simulink model "frbd_64ch_600mhz2"  (R2013b)
settings: Solver=FixedStepDiscrete  SolverMode=SingleTasking  StartTime=0.0  StopTime=10.0  RelTol=1e-3
undefined symbols (not defined in the file or in its folder): pfb_coeff_gen_calc
libraries: xbsIndex_r4 x13876, casper_library_misc x58, casper_library_delays x32, dspsigops x16, casper_library_pfbs x2, xps_library x1
(part 16 of 138)

== system frbd_64ch_600mhz2/ACC7/mem ==
  note: Undo address
      | manipulation for
      | simulated data
  note: Undo data manipulation on way in and redo on way out for simulated data
  In1 : Inport
  In2 : Inport  Port=2
  In3 : Inport  Port=3
  Disregard Subsystem : xbsIndex_r4/Disregard Subsystem  Tag=discardX  block_type=disregard
  calc_add : Subsystem  mask{data_width=32, addr_width=10, sample_rate=sample_rate}
      mask prompts: data_width "data width"; addr_width "address width"; sample_rate "sample rate"
  ram : xbsIndex_r4/Single Port RAM  depth=2^addr_width  initVector=init_vals  distributed_mem=Block RAM  write_mode=Read After Write  rst=off  init_reg=0  en=off  latency=3  dbl_ovrd=off  optimize=Area  block_type=spram
  sim_addr : xbsIndex_r4/Gateway In  gui_display_data_type=Fixed-point  arith_type=Unsigned  n_bits=addr_width  bin_pt=0  preci_type=Single  exp_width=8  frac_width=24  quantization=Truncate  overflow=Wrap  period=sample_rate  dbl_ovrd=off  timing_constraint=None  locs_specified=off  LOCs={}  UseAsADC=off  ADCChannel='1'  inherit_from_input=off  hdl_port=on  block_type=gatewayin
      settings: infoedit="Gateway in block.  Converts inputs of type Simulink integer, double and fixed point to  Xilinx fixed point type.<br><br>Hardware notes:  In hardware these blocks become top level input ports."  xl_area=[0, 0, 0, 0, 0, 0, 0]  sginterface={'Nallatech'=>{'xdspkit'=>{'non_memory_mapped_port'=>'sim_addr'}},'Xilinx'=>{'jtaghwcosim'=>{'non_memory_mapped_port'=>'sim_addr'},'xdspkit'=>{'non_memory_mapped_port'=>'sim_addr'}}}
  sim_data_in : xbsIndex_r4/Gateway In  gui_display_data_type=Fixed-point  arith_type=Unsigned  n_bits=32  bin_pt=0  preci_type=Single  exp_width=8  frac_width=24  quantization=Truncate  overflow=Wrap  period=sample_rate  dbl_ovrd=off  timing_constraint=None  locs_specified=off  LOCs={}  UseAsADC=off  ADCChannel='1'  inherit_from_input=off  hdl_port=on  block_type=gatewayin
      settings: xl_area=[0, 0, 0, 0, 0, 0, 0]  sginterface={'Nallatech'=>{'xdspkit'=>{'non_memory_mapped_port'=>'sim_data_in'}},'Xilinx'=>{'jtaghwcosim'=>{'non_memory_mapped_port'=>'sim_data_in'},'xdspkit'=>{'non_memory_mapped_port'=>'sim_data_in'}}}
  sim_data_out : xbsIndex_r4/Gateway Out  inherit_from_input=off  hdl_port=on  timing_constraint=None  locs_specified=off  LOCs={'B21','B22','A22','B23','B19','C19','A20','A21','A23','B24','A24','A25','E18','D18','C18','B18'}  UseAsDAC=off  DACChannel='1'  block_type=gatewayout
      settings: infoedit="Gateway out block.  Converts Xilinx fixed point inputs into ouputs of type Simulink integer, double, or fixed point.<P><P>Hardware notes:  In hardware these blocks become top level output ports or are discarded, depending on how they are configured."  xl_area=[0, 0, 0, 0, 0, 0, 0]  sginterface={'Nallatech'=>{'xdspkit'=>{'non_memory_mapped_port'=>'sim_data_out'}},'Xilinx'=>{'jtaghwcosim'=>{'non_memory_mapped_port'=>'sim_data_out'},'xdspkit'=>{'non_memory_mapped_port'=>'sim_data_out'}}}
  sim_munge_in : Subsystem  AncestorBlock=casper_library_flow_control/munge  mask(munge){divisions=1, div_size=32, order=[0], arith_type_out=Unsigned, bin_pt_out=0}
      mask prompts: divisions "Number of divisions"; div_size "Division size (bits)"; order "Division packing order"; arith_type_out "Output arithmetic type"; bin_pt_out "Output binary point"
      mask help: Splits an input bus into the specified number of divisions and then recombines them in the order specified (most significant division = 0,least = number divisions-1)
      mask init:
      | munge_init(gcb, ...
      |     'divisions', divisions, ...
      |     'div_size', div_size, ...
      |     'order', order, ...
      |     'arith_type_out', arith_type_out, ...
      |     'bin_pt_out', bin_pt_out);
      settings: AttributesFormatString=|
      | split:32
      | join:0
      | Unsigned [32,0]
      mask TypeOptions arith_type_out: Unsigned | Signed  (2's comp) | Floating-point
  sim_munge_out : Subsystem  AncestorBlock=casper_library_flow_control/munge  mask(munge){divisions=1, div_size=32, order=[0], arith_type_out=Unsigned, bin_pt_out=0}
      mask prompts: divisions "Number of divisions"; div_size "Division size (bits)"; order "Division packing order"; arith_type_out "Output arithmetic type"; bin_pt_out "Output binary point"
      mask help: Splits an input bus into the specified number of divisions and then recombines them in the order specified (most significant division = 0,least = number divisions-1)
      mask init:
      | munge_init(gcb, ...
      |     'divisions', divisions, ...
      |     'div_size', div_size, ...
      |     'order', order, ...
      |     'arith_type_out', arith_type_out, ...
      |     'bin_pt_out', bin_pt_out);
      settings: AttributesFormatString=|
      | split:32
      | join:0
      | Unsigned [32,0]
      mask TypeOptions arith_type_out: Unsigned | Signed  (2's comp) | Floating-point
  sim_we : xbsIndex_r4/Gateway In  gui_display_data_type=Fixed-point  arith_type=Boolean  n_bits=1  bin_pt=0  preci_type=Single  exp_width=8  frac_width=24  quantization=Truncate  overflow=Wrap  period=sample_rate  dbl_ovrd=off  timing_constraint=None  locs_specified=off  LOCs={}  UseAsADC=off  ADCChannel='1'  inherit_from_input=off  hdl_port=on  block_type=gatewayin
      settings: infoedit="Gateway in block.  Converts inputs of type Simulink integer, double and fixed point to  Xilinx fixed point type.<br><br>Hardware notes:  In hardware these blocks become top level input ports."  xl_area=[0, 0, 0, 0, 0, 0, 0]  sginterface={'Nallatech'=>{'xdspkit'=>{'non_memory_mapped_port'=>'sim_we'}},'Xilinx'=>{'jtaghwcosim'=>{'non_memory_mapped_port'=>'sim_we'},'xdspkit'=>{'non_memory_mapped_port'=>'sim_we'}}}
  Out1 : Outport
  wires:
  sim_munge_in/1(dout) -> ram/2
  ram/1 -> sim_munge_out/1(din)
  sim_we/1 -> ram/3
  sim_data_in/1 -> sim_munge_in/1(din)
  sim_addr/1 -> calc_add/1(in)
  In3/1 -> sim_we/1
  sim_data_out/1 -> Out1/1
  In2/1 -> sim_data_in/1
  In1/1 -> sim_addr/1
  sim_munge_out/1(dout) -> sim_data_out/1
  calc_add/1(out) -> ram/1

== system frbd_64ch_600mhz2/ACC7/munge_in ==
  din : Inport
  reinterpret_out : xbsIndex_r4/Reinterpret  force_arith_type=on  arith_type=Unsigned  force_bin_pt=on  bin_pt=0  block_type=reinterpret
  dout : Outport
  wires:
  reinterpret_out/1 -> dout/1
  din/1 -> reinterpret_out/1

== system frbd_64ch_600mhz2/ACC7/munge_out ==
  din : Inport
  reinterpret_out : xbsIndex_r4/Reinterpret  force_arith_type=on  arith_type=Unsigned  force_bin_pt=on  bin_pt=0  block_type=reinterpret
  dout : Outport
  wires:
  reinterpret_out/1 -> dout/1
  din/1 -> reinterpret_out/1

== system frbd_64ch_600mhz2/ACC8/calc_add ==
  note: Use behavioural HDL
      | so that gets optimised
      | to minimum logic
  note: If reading/writing words
      | smaller than 32 bits,
      | change address so
      | that addressing is
      | big endian instead of
      | little, otherwise
      | pass through
  in : Inport
  add_sub : xbsIndex_r4/AddSub  mode=Subtraction  use_carryin=off  use_carryout=off  en=off  latency=0  precision=User Defined  arith_type=Unsigned  n_bits=max(1, log2(32/data_width))  bin_pt=0  quantization=Truncate  overflow=Wrap  dbl_ovrd=off  use_behavioral_HDL=on  hw_selection=Fabric  pipelined=off  block_type=addsub
  concat : xbsIndex_r4/Concat  num_inputs=2  dbl_ovrd=off  block_type=concat
  const : xbsIndex_r4/Constant  const=max(0, 32/data_width-1)  gui_display_data_type=Fixed-point  arith_type=Unsigned  n_bits=max(1, log2(32/data_width))  bin_pt=0  preci_type=Single  exp_width=8  frac_width=24  explicit_period=on  period=sample_rate  equ=P=C  opselect=C  inp2=PCIN>>17  opr=+  inp1=P  carry=CIN  dbl_ovrd=off  block_type=constant
      settings: block_version=11.4
  convert_addr : xbsIndex_r4/Convert  gui_display_data_type=Fixed-point  arith_type=Unsigned  n_bits=addr_width  bin_pt=0  float_type=Single  exp_bits=8  fraction_bits=24  quantization=Truncate  overflow=Wrap  en=off  latency=0  dbl_ovrd=off  pipeline=off  block_type=convert
      settings: xl_area=[0, 0, 0, 0, 0, 0, 0]
  lsw : xbsIndex_r4/Slice  nbits=max(1, log2(32/data_width))  boolean_output=off  mode=Lower Bit Location + Width  bit1=0  base1=MSB of Input  bit0=0  base0=LSB of Input  dbl_ovrd=off  block_type=slice
  manipulate : xbsIndex_r4/Constant  const=min(1, floor(32/data_width) - 1)  gui_display_data_type=Fixed-point  arith_type=Unsigned  n_bits=1  bin_pt=0  preci_type=Single  exp_width=8  frac_width=24  explicit_period=on  period=sample_rate  equ=P=C  opselect=C  inp2=PCIN>>17  opr=+  inp1=P  carry=CIN  dbl_ovrd=off  block_type=constant
      settings: block_version=11.4
  msw : xbsIndex_r4/Slice  nbits=addr_width - max(1, log2(32/data_width))  boolean_output=off  mode=Upper Bit Location + Width  bit1=0  base1=MSB of Input  bit0=0  base0=LSB of Input  dbl_ovrd=off  block_type=slice
  mux : xbsIndex_r4/Mux  inputs=2  en=off  latency=0  precision=Full  arith_type=Unsigned  n_bits=16  bin_pt=14  quantization=Truncate  overflow=Wrap  dbl_ovrd=off  block_type=mux
      settings: block_version=11.4
  out : Outport
  wires:
  convert_addr/1 -> mux/2, msw/1, lsw/1
  const/1 -> add_sub/1
  lsw/1 -> add_sub/2
  mux/1 -> out/1
  manipulate/1 -> mux/1
  concat/1 -> mux/3
  msw/1 -> concat/1
  add_sub/1 -> concat/2
  in/1 -> convert_addr/1

== system frbd_64ch_600mhz2/ACC8/mem ==
  note: Undo data manipulation on way in and redo on way out for simulated data
  note: Undo address
      | manipulation for
      | simulated data
  In1 : Inport
  In2 : Inport  Port=2
  In3 : Inport  Port=3
  Disregard Subsystem : xbsIndex_r4/Disregard Subsystem  Tag=discardX  block_type=disregard
  calc_add : Subsystem  mask{data_width=32, addr_width=10, sample_rate=sample_rate}
      mask prompts: data_width "data width"; addr_width "address width"; sample_rate "sample rate"
  ram : xbsIndex_r4/Single Port RAM  depth=2^addr_width  initVector=init_vals  distributed_mem=Block RAM  write_mode=Read After Write  rst=off  init_reg=0  en=off  latency=3  dbl_ovrd=off  optimize=Area  block_type=spram
  sim_addr : xbsIndex_r4/Gateway In  gui_display_data_type=Fixed-point  arith_type=Unsigned  n_bits=addr_width  bin_pt=0  preci_type=Single  exp_width=8  frac_width=24  quantization=Truncate  overflow=Wrap  period=sample_rate  dbl_ovrd=off  timing_constraint=None  locs_specified=off  LOCs={}  UseAsADC=off  ADCChannel='1'  inherit_from_input=off  hdl_port=on  block_type=gatewayin
      settings: infoedit="Gateway in block.  Converts inputs of type Simulink integer, double and fixed point to  Xilinx fixed point type.<br><br>Hardware notes:  In hardware these blocks become top level input ports."  xl_area=[0, 0, 0, 0, 0, 0, 0]  sginterface={'Nallatech'=>{'xdspkit'=>{'non_memory_mapped_port'=>'sim_addr'}},'Xilinx'=>{'jtaghwcosim'=>{'non_memory_mapped_port'=>'sim_addr'},'xdspkit'=>{'non_memory_mapped_port'=>'sim_addr'}}}
  sim_data_in : xbsIndex_r4/Gateway In  gui_display_data_type=Fixed-point  arith_type=Unsigned  n_bits=32  bin_pt=0  preci_type=Single  exp_width=8  frac_width=24  quantization=Truncate  overflow=Wrap  period=sample_rate  dbl_ovrd=off  timing_constraint=None  locs_specified=off  LOCs={}  UseAsADC=off  ADCChannel='1'  inherit_from_input=off  hdl_port=on  block_type=gatewayin
      settings: xl_area=[0, 0, 0, 0, 0, 0, 0]  sginterface={'Nallatech'=>{'xdspkit'=>{'non_memory_mapped_port'=>'sim_data_in'}},'Xilinx'=>{'jtaghwcosim'=>{'non_memory_mapped_port'=>'sim_data_in'},'xdspkit'=>{'non_memory_mapped_port'=>'sim_data_in'}}}
  sim_data_out : xbsIndex_r4/Gateway Out  inherit_from_input=off  hdl_port=on  timing_constraint=None  locs_specified=off  LOCs={'B21','B22','A22','B23','B19','C19','A20','A21','A23','B24','A24','A25','E18','D18','C18','B18'}  UseAsDAC=off  DACChannel='1'  block_type=gatewayout
      settings: infoedit="Gateway out block.  Converts Xilinx fixed point inputs into ouputs of type Simulink integer, double, or fixed point.<P><P>Hardware notes:  In hardware these blocks become top level output ports or are discarded, depending on how they are configured."  xl_area=[0, 0, 0, 0, 0, 0, 0]  sginterface={'Nallatech'=>{'xdspkit'=>{'non_memory_mapped_port'=>'sim_data_out'}},'Xilinx'=>{'jtaghwcosim'=>{'non_memory_mapped_port'=>'sim_data_out'},'xdspkit'=>{'non_memory_mapped_port'=>'sim_data_out'}}}
  sim_munge_in : Subsystem  AncestorBlock=casper_library_flow_control/munge  mask(munge){divisions=1, div_size=32, order=[0], arith_type_out=Unsigned, bin_pt_out=0}
      mask prompts: divisions "Number of divisions"; div_size "Division size (bits)"; order "Division packing order"; arith_type_out "Output arithmetic type"; bin_pt_out "Output binary point"
      mask help: Splits an input bus into the specified number of divisions and then recombines them in the order specified (most significant division = 0,least = number divisions-1)
      mask init:
      | munge_init(gcb, ...
      |     'divisions', divisions, ...
      |     'div_size', div_size, ...
      |     'order', order, ...
      |     'arith_type_out', arith_type_out, ...
      |     'bin_pt_out', bin_pt_out);
      settings: AttributesFormatString=|
      | split:32
      | join:0
      | Unsigned [32,0]
      mask TypeOptions arith_type_out: Unsigned | Signed  (2's comp) | Floating-point
  sim_munge_out : Subsystem  AncestorBlock=casper_library_flow_control/munge  mask(munge){divisions=1, div_size=32, order=[0], arith_type_out=Unsigned, bin_pt_out=0}
      mask prompts: divisions "Number of divisions"; div_size "Division size (bits)"; order "Division packing order"; arith_type_out "Output arithmetic type"; bin_pt_out "Output binary point"
      mask help: Splits an input bus into the specified number of divisions and then recombines them in the order specified (most significant division = 0,least = number divisions-1)
      mask init:
      | munge_init(gcb, ...
      |     'divisions', divisions, ...
      |     'div_size', div_size, ...
      |     'order', order, ...
      |     'arith_type_out', arith_type_out, ...
      |     'bin_pt_out', bin_pt_out);
      settings: AttributesFormatString=|
      | split:32
      | join:0
      | Unsigned [32,0]
      mask TypeOptions arith_type_out: Unsigned | Signed  (2's comp) | Floating-point
  sim_we : xbsIndex_r4/Gateway In  gui_display_data_type=Fixed-point  arith_type=Boolean  n_bits=1  bin_pt=0  preci_type=Single  exp_width=8  frac_width=24  quantization=Truncate  overflow=Wrap  period=sample_rate  dbl_ovrd=off  timing_constraint=None  locs_specified=off  LOCs={}  UseAsADC=off  ADCChannel='1'  inherit_from_input=off  hdl_port=on  block_type=gatewayin
      settings: infoedit="Gateway in block.  Converts inputs of type Simulink integer, double and fixed point to  Xilinx fixed point type.<br><br>Hardware notes:  In hardware these blocks become top level input ports."  xl_area=[0, 0, 0, 0, 0, 0, 0]  sginterface={'Nallatech'=>{'xdspkit'=>{'non_memory_mapped_port'=>'sim_we'}},'Xilinx'=>{'jtaghwcosim'=>{'non_memory_mapped_port'=>'sim_we'},'xdspkit'=>{'non_memory_mapped_port'=>'sim_we'}}}
  Out1 : Outport
  wires:
  calc_add/1(out) -> ram/1
  sim_munge_out/1(dout) -> sim_data_out/1
  In1/1 -> sim_addr/1
  In2/1 -> sim_data_in/1
  sim_data_out/1 -> Out1/1
  In3/1 -> sim_we/1
  sim_addr/1 -> calc_add/1(in)
  sim_data_in/1 -> sim_munge_in/1(din)
  sim_we/1 -> ram/3
  ram/1 -> sim_munge_out/1(din)
  sim_munge_in/1(dout) -> ram/2

== system frbd_64ch_600mhz2/ACC8/munge_in ==
  din : Inport
  reinterpret_out : xbsIndex_r4/Reinterpret  force_arith_type=on  arith_type=Unsigned  force_bin_pt=on  bin_pt=0  block_type=reinterpret
  dout : Outport
  wires:
  din/1 -> reinterpret_out/1
  reinterpret_out/1 -> dout/1

== system frbd_64ch_600mhz2/ACC8/munge_out ==
  din : Inport
  reinterpret_out : xbsIndex_r4/Reinterpret  force_arith_type=on  arith_type=Unsigned  force_bin_pt=on  bin_pt=0  block_type=reinterpret
  dout : Outport
  wires:
  din/1 -> reinterpret_out/1
  reinterpret_out/1 -> dout/1

== system frbd_64ch_600mhz2/ACC9/calc_add ==
  note: Use behavioural HDL
      | so that gets optimised
      | to minimum logic
  note: If reading/writing words
      | smaller than 32 bits,
      | change address so
      | that addressing is
      | big endian instead of
      | little, otherwise
      | pass through
  in : Inport
  add_sub : xbsIndex_r4/AddSub  mode=Subtraction  use_carryin=off  use_carryout=off  en=off  latency=0  precision=User Defined  arith_type=Unsigned  n_bits=max(1, log2(32/data_width))  bin_pt=0  quantization=Truncate  overflow=Wrap  dbl_ovrd=off  use_behavioral_HDL=on  hw_selection=Fabric  pipelined=off  block_type=addsub
  concat : xbsIndex_r4/Concat  num_inputs=2  dbl_ovrd=off  block_type=concat
  const : xbsIndex_r4/Constant  const=max(0, 32/data_width-1)  gui_display_data_type=Fixed-point  arith_type=Unsigned  n_bits=max(1, log2(32/data_width))  bin_pt=0  preci_type=Single  exp_width=8  frac_width=24  explicit_period=on  period=sample_rate  equ=P=C  opselect=C  inp2=PCIN>>17  opr=+  inp1=P  carry=CIN  dbl_ovrd=off  block_type=constant
      settings: block_version=11.4
  convert_addr : xbsIndex_r4/Convert  gui_display_data_type=Fixed-point  arith_type=Unsigned  n_bits=addr_width  bin_pt=0  float_type=Single  exp_bits=8  fraction_bits=24  quantization=Truncate  overflow=Wrap  en=off  latency=0  dbl_ovrd=off  pipeline=off  block_type=convert
      settings: xl_area=[0, 0, 0, 0, 0, 0, 0]
  lsw : xbsIndex_r4/Slice  nbits=max(1, log2(32/data_width))  boolean_output=off  mode=Lower Bit Location + Width  bit1=0  base1=MSB of Input  bit0=0  base0=LSB of Input  dbl_ovrd=off  block_type=slice
  manipulate : xbsIndex_r4/Constant  const=min(1, floor(32/data_width) - 1)  gui_display_data_type=Fixed-point  arith_type=Unsigned  n_bits=1  bin_pt=0  preci_type=Single  exp_width=8  frac_width=24  explicit_period=on  period=sample_rate  equ=P=C  opselect=C  inp2=PCIN>>17  opr=+  inp1=P  carry=CIN  dbl_ovrd=off  block_type=constant
      settings: block_version=11.4
  msw : xbsIndex_r4/Slice  nbits=addr_width - max(1, log2(32/data_width))  boolean_output=off  mode=Upper Bit Location + Width  bit1=0  base1=MSB of Input  bit0=0  base0=LSB of Input  dbl_ovrd=off  block_type=slice
  mux : xbsIndex_r4/Mux  inputs=2  en=off  latency=0  precision=Full  arith_type=Unsigned  n_bits=16  bin_pt=14  quantization=Truncate  overflow=Wrap  dbl_ovrd=off  block_type=mux
      settings: block_version=11.4
  out : Outport
  wires:
  convert_addr/1 -> mux/2, msw/1, lsw/1
  const/1 -> add_sub/1
  lsw/1 -> add_sub/2
  mux/1 -> out/1
  manipulate/1 -> mux/1
  concat/1 -> mux/3
  msw/1 -> concat/1
  add_sub/1 -> concat/2
  in/1 -> convert_addr/1

== system frbd_64ch_600mhz2/ACC9/mem ==
  note: Undo data manipulation on way in and redo on way out for simulated data
  note: Undo address
      | manipulation for
      | simulated data
  In1 : Inport
  In2 : Inport  Port=2
  In3 : Inport  Port=3
  Disregard Subsystem : xbsIndex_r4/Disregard Subsystem  Tag=discardX  block_type=disregard
  calc_add : Subsystem  mask{data_width=32, addr_width=10, sample_rate=sample_rate}
      mask prompts: data_width "data width"; addr_width "address width"; sample_rate "sample rate"
  ram : xbsIndex_r4/Single Port RAM  depth=2^addr_width  initVector=init_vals  distributed_mem=Block RAM  write_mode=Read After Write  rst=off  init_reg=0  en=off  latency=3  dbl_ovrd=off  optimize=Area  block_type=spram
  sim_addr : xbsIndex_r4/Gateway In  gui_display_data_type=Fixed-point  arith_type=Unsigned  n_bits=addr_width  bin_pt=0  preci_type=Single  exp_width=8  frac_width=24  quantization=Truncate  overflow=Wrap  period=sample_rate  dbl_ovrd=off  timing_constraint=None  locs_specified=off  LOCs={}  UseAsADC=off  ADCChannel='1'  inherit_from_input=off  hdl_port=on  block_type=gatewayin
      settings: infoedit="Gateway in block.  Converts inputs of type Simulink integer, double and fixed point to  Xilinx fixed point type.<br><br>Hardware notes:  In hardware these blocks become top level input ports."  xl_area=[0, 0, 0, 0, 0, 0, 0]  sginterface={'Nallatech'=>{'xdspkit'=>{'non_memory_mapped_port'=>'sim_addr'}},'Xilinx'=>{'jtaghwcosim'=>{'non_memory_mapped_port'=>'sim_addr'},'xdspkit'=>{'non_memory_mapped_port'=>'sim_addr'}}}
  sim_data_in : xbsIndex_r4/Gateway In  gui_display_data_type=Fixed-point  arith_type=Unsigned  n_bits=32  bin_pt=0  preci_type=Single  exp_width=8  frac_width=24  quantization=Truncate  overflow=Wrap  period=sample_rate  dbl_ovrd=off  timing_constraint=None  locs_specified=off  LOCs={}  UseAsADC=off  ADCChannel='1'  inherit_from_input=off  hdl_port=on  block_type=gatewayin
      settings: xl_area=[0, 0, 0, 0, 0, 0, 0]  sginterface={'Nallatech'=>{'xdspkit'=>{'non_memory_mapped_port'=>'sim_data_in'}},'Xilinx'=>{'jtaghwcosim'=>{'non_memory_mapped_port'=>'sim_data_in'},'xdspkit'=>{'non_memory_mapped_port'=>'sim_data_in'}}}
  sim_data_out : xbsIndex_r4/Gateway Out  inherit_from_input=off  hdl_port=on  timing_constraint=None  locs_specified=off  LOCs={'B21','B22','A22','B23','B19','C19','A20','A21','A23','B24','A24','A25','E18','D18','C18','B18'}  UseAsDAC=off  DACChannel='1'  block_type=gatewayout
      settings: infoedit="Gateway out block.  Converts Xilinx fixed point inputs into ouputs of type Simulink integer, double, or fixed point.<P><P>Hardware notes:  In hardware these blocks become top level output ports or are discarded, depending on how they are configured."  xl_area=[0, 0, 0, 0, 0, 0, 0]  sginterface={'Nallatech'=>{'xdspkit'=>{'non_memory_mapped_port'=>'sim_data_out'}},'Xilinx'=>{'jtaghwcosim'=>{'non_memory_mapped_port'=>'sim_data_out'},'xdspkit'=>{'non_memory_mapped_port'=>'sim_data_out'}}}
  sim_munge_in : Subsystem  AncestorBlock=casper_library_flow_control/munge  mask(munge){divisions=1, div_size=32, order=[0], arith_type_out=Unsigned, bin_pt_out=0}
      mask prompts: divisions "Number of divisions"; div_size "Division size (bits)"; order "Division packing order"; arith_type_out "Output arithmetic type"; bin_pt_out "Output binary point"
      mask help: Splits an input bus into the specified number of divisions and then recombines them in the order specified (most significant division = 0,least = number divisions-1)
      mask init:
      | munge_init(gcb, ...
      |     'divisions', divisions, ...
      |     'div_size', div_size, ...
      |     'order', order, ...
      |     'arith_type_out', arith_type_out, ...
      |     'bin_pt_out', bin_pt_out);
      settings: AttributesFormatString=|
      | split:32
      | join:0
      | Unsigned [32,0]
      mask TypeOptions arith_type_out: Unsigned | Signed  (2's comp) | Floating-point
  sim_munge_out : Subsystem  AncestorBlock=casper_library_flow_control/munge  mask(munge){divisions=1, div_size=32, order=[0], arith_type_out=Unsigned, bin_pt_out=0}
      mask prompts: divisions "Number of divisions"; div_size "Division size (bits)"; order "Division packing order"; arith_type_out "Output arithmetic type"; bin_pt_out "Output binary point"
      mask help: Splits an input bus into the specified number of divisions and then recombines them in the order specified (most significant division = 0,least = number divisions-1)
      mask init:
      | munge_init(gcb, ...
      |     'divisions', divisions, ...
      |     'div_size', div_size, ...
      |     'order', order, ...
      |     'arith_type_out', arith_type_out, ...
      |     'bin_pt_out', bin_pt_out);
      settings: AttributesFormatString=|
      | split:32
      | join:0
      | Unsigned [32,0]
      mask TypeOptions arith_type_out: Unsigned | Signed  (2's comp) | Floating-point
  sim_we : xbsIndex_r4/Gateway In  gui_display_data_type=Fixed-point  arith_type=Boolean  n_bits=1  bin_pt=0  preci_type=Single  exp_width=8  frac_width=24  quantization=Truncate  overflow=Wrap  period=sample_rate  dbl_ovrd=off  timing_constraint=None  locs_specified=off  LOCs={}  UseAsADC=off  ADCChannel='1'  inherit_from_input=off  hdl_port=on  block_type=gatewayin
      settings: infoedit="Gateway in block.  Converts inputs of type Simulink integer, double and fixed point to  Xilinx fixed point type.<br><br>Hardware notes:  In hardware these blocks become top level input ports."  xl_area=[0, 0, 0, 0, 0, 0, 0]  sginterface={'Nallatech'=>{'xdspkit'=>{'non_memory_mapped_port'=>'sim_we'}},'Xilinx'=>{'jtaghwcosim'=>{'non_memory_mapped_port'=>'sim_we'},'xdspkit'=>{'non_memory_mapped_port'=>'sim_we'}}}
  Out1 : Outport
  wires:
  calc_add/1(out) -> ram/1
  sim_munge_out/1(dout) -> sim_data_out/1
  In1/1 -> sim_addr/1
  In2/1 -> sim_data_in/1
  sim_data_out/1 -> Out1/1
  In3/1 -> sim_we/1
  sim_addr/1 -> calc_add/1(in)
  sim_data_in/1 -> sim_munge_in/1(din)
  sim_we/1 -> ram/3
  ram/1 -> sim_munge_out/1(din)
  sim_munge_in/1(dout) -> ram/2

== system frbd_64ch_600mhz2/ACC9/munge_in ==
  din : Inport
  reinterpret_out : xbsIndex_r4/Reinterpret  force_arith_type=on  arith_type=Unsigned  force_bin_pt=on  bin_pt=0  block_type=reinterpret
  dout : Outport
  wires:
  din/1 -> reinterpret_out/1
  reinterpret_out/1 -> dout/1

== system frbd_64ch_600mhz2/ACC9/munge_out ==
  din : Inport
  reinterpret_out : xbsIndex_r4/Reinterpret  force_arith_type=on  arith_type=Unsigned  force_bin_pt=on  bin_pt=0  block_type=reinterpret
  dout : Outport
  wires:
  din/1 -> reinterpret_out/1
  reinterpret_out/1 -> dout/1

== system frbd_64ch_600mhz2/Parallel_Dedispersor_v1/Dedispersor_v2_1 ==
  Data : Inport
  Valid : Inport  Port=2
  Counter : xbsIndex_r4/Counter  cnt_type=Free Running  cnt_to=Inf  operation=Up  start_count=0  cnt_by_val=1  arith_type=Unsigned  n_bits=4  bin_pt=0  load_pin=off  rst=off  en=on  explicit_period=on  period=1  dbl_ovrd=off  use_behavioral_HDL=off  implementation=Fabric  block_type=counter
  Mux : xbsIndex_r4/Mux  inputs=16  en=off  latency=0  precision=Full  arith_type=Unsigned  n_bits=16  bin_pt=14  quantization=Truncate  overflow=Wrap  dbl_ovrd=off  block_type=mux
  detector_block_v2 : Subsystem  AncestorBlock=honestlibrary/detector_block_v2  mask(Basic block for FRB detection){chn=0, lat=1, nbits=4}
      mask prompts: chn "Channel"; lat "Latency"; nbits "Number of Bits (Counter)"
      mask help:
      | Delays a certain channel a number of latency clock cycles, according to the fixed DM table.
      | This version incorporates an internal counter (nbits) to know when store or give a certain value.
      mask init:
      | detector_block_init_v2(gcb,'chn',chn,'lat',lat,'nbits',nbits)
      settings: AttributesFormatString=Channel: 0, Delay: 1
  detector_block_v21 : Subsystem  AncestorBlock=honestlibrary/detector_block_v2  mask(Basic block for FRB detection){chn=1, lat=12, nbits=4}
      mask prompts: chn "Channel"; lat "Latency"; nbits "Number of Bits (Counter)"
      mask help:
      | Delays a certain channel a number of latency clock cycles, according to the fixed DM table.
      | This version incorporates an internal counter (nbits) to know when store or give a certain value.
      mask init:
      | detector_block_init_v2(gcb,'chn',chn,'lat',lat,'nbits',nbits)
      settings: AttributesFormatString=Channel: 1, Delay: 12
  detector_block_v210 : Subsystem  AncestorBlock=honestlibrary/detector_block_v2  mask(Basic block for FRB detection){chn=10, lat=89, nbits=4}
      mask prompts: chn "Channel"; lat "Latency"; nbits "Number of Bits (Counter)"
      mask help:
      | Delays a certain channel a number of latency clock cycles, according to the fixed DM table.
      | This version incorporates an internal counter (nbits) to know when store or give a certain value.
      mask init:
      | detector_block_init_v2(gcb,'chn',chn,'lat',lat,'nbits',nbits)
      settings: AttributesFormatString=Channel: 10, Delay: 89
  detector_block_v211 : Subsystem  AncestorBlock=honestlibrary/detector_block_v2  mask(Basic block for FRB detection){chn=11, lat=95, nbits=4}
      mask prompts: chn "Channel"; lat "Latency"; nbits "Number of Bits (Counter)"
      mask help:
      | Delays a certain channel a number of latency clock cycles, according to the fixed DM table.
      | This version incorporates an internal counter (nbits) to know when store or give a certain value.
      mask init:
      | detector_block_init_v2(gcb,'chn',chn,'lat',lat,'nbits',nbits)
      settings: AttributesFormatString=Channel: 11, Delay: 95
  detector_block_v212 : Subsystem  AncestorBlock=honestlibrary/detector_block_v2  mask(Basic block for FRB detection){chn=12, lat=100, nbits=4}
      mask prompts: chn "Channel"; lat "Latency"; nbits "Number of Bits (Counter)"
      mask help:
      | Delays a certain channel a number of latency clock cycles, according to the fixed DM table.
      | This version incorporates an internal counter (nbits) to know when store or give a certain value.
      mask init:
      | detector_block_init_v2(gcb,'chn',chn,'lat',lat,'nbits',nbits)
      settings: AttributesFormatString=Channel: 12, Delay: 100
  detector_block_v213 : Subsystem  AncestorBlock=honestlibrary/detector_block_v2  mask(Basic block for FRB detection){chn=13, lat=105, nbits=4}
      mask prompts: chn "Channel"; lat "Latency"; nbits "Number of Bits (Counter)"
      mask help:
      | Delays a certain channel a number of latency clock cycles, according to the fixed DM table.
      | This version incorporates an internal counter (nbits) to know when store or give a certain value.
      mask init:
      | detector_block_init_v2(gcb,'chn',chn,'lat',lat,'nbits',nbits)
      settings: AttributesFormatString=Channel: 13, Delay: 105
  detector_block_v214 : Subsystem  AncestorBlock=honestlibrary/detector_block_v2  mask(Basic block for FRB detection){chn=14, lat=110, nbits=4}
      mask prompts: chn "Channel"; lat "Latency"; nbits "Number of Bits (Counter)"
      mask help:
      | Delays a certain channel a number of latency clock cycles, according to the fixed DM table.
      | This version incorporates an internal counter (nbits) to know when store or give a certain value.
      mask init:
      | detector_block_init_v2(gcb,'chn',chn,'lat',lat,'nbits',nbits)
      settings: AttributesFormatString=Channel: 14, Delay: 110
  detector_block_v215 : Subsystem  AncestorBlock=honestlibrary/detector_block_v2  mask(Basic block for FRB detection){chn=15, lat=114, nbits=4}
      mask prompts: chn "Channel"; lat "Latency"; nbits "Number of Bits (Counter)"
      mask help:
      | Delays a certain channel a number of latency clock cycles, according to the fixed DM table.
      | This version incorporates an internal counter (nbits) to know when store or give a certain value.
      mask init:
      | detector_block_init_v2(gcb,'chn',chn,'lat',lat,'nbits',nbits)
      settings: AttributesFormatString=Channel: 15, Delay: 114
  detector_block_v22 : Subsystem  AncestorBlock=honestlibrary/detector_block_v2  mask(Basic block for FRB detection){chn=2, lat=23, nbits=4}
      mask prompts: chn "Channel"; lat "Latency"; nbits "Number of Bits (Counter)"
      mask help:
      | Delays a certain channel a number of latency clock cycles, according to the fixed DM table.
      | This version incorporates an internal counter (nbits) to know when store or give a certain value.
      mask init:
      | detector_block_init_v2(gcb,'chn',chn,'lat',lat,'nbits',nbits)
      settings: AttributesFormatString=Channel: 2, Delay: 23
  detector_block_v23 : Subsystem  AncestorBlock=honestlibrary/detector_block_v2  mask(Basic block for FRB detection){chn=3, lat=34, nbits=4}
      mask prompts: chn "Channel"; lat "Latency"; nbits "Number of Bits (Counter)"
      mask help:
      | Delays a certain channel a number of latency clock cycles, according to the fixed DM table.
      | This version incorporates an internal counter (nbits) to know when store or give a certain value.
      mask init:
      | detector_block_init_v2(gcb,'chn',chn,'lat',lat,'nbits',nbits)
      settings: AttributesFormatString=Channel: 3, Delay: 34
  detector_block_v24 : Subsystem  AncestorBlock=honestlibrary/detector_block_v2  mask(Basic block for FRB detection){chn=4, lat=44, nbits=4}
      mask prompts: chn "Channel"; lat "Latency"; nbits "Number of Bits (Counter)"
      mask help:
      | Delays a certain channel a number of latency clock cycles, according to the fixed DM table.
      | This version incorporates an internal counter (nbits) to know when store or give a certain value.
      mask init:
      | detector_block_init_v2(gcb,'chn',chn,'lat',lat,'nbits',nbits)
      settings: AttributesFormatString=Channel: 4, Delay: 44
  detector_block_v25 : Subsystem  AncestorBlock=honestlibrary/detector_block_v2  mask(Basic block for FRB detection){chn=5, lat=53, nbits=4}
      mask prompts: chn "Channel"; lat "Latency"; nbits "Number of Bits (Counter)"
      mask help:
      | Delays a certain channel a number of latency clock cycles, according to the fixed DM table.
      | This version incorporates an internal counter (nbits) to know when store or give a certain value.
      mask init:
      | detector_block_init_v2(gcb,'chn',chn,'lat',lat,'nbits',nbits)
      settings: AttributesFormatString=Channel: 5, Delay: 53
  detector_block_v26 : Subsystem  AncestorBlock=honestlibrary/detector_block_v2  mask(Basic block for FRB detection){chn=6, lat=61, nbits=4}
      mask prompts: chn "Channel"; lat "Latency"; nbits "Number of Bits (Counter)"
      mask help:
      | Delays a certain channel a number of latency clock cycles, according to the fixed DM table.
      | This version incorporates an internal counter (nbits) to know when store or give a certain value.
      mask init:
      | detector_block_init_v2(gcb,'chn',chn,'lat',lat,'nbits',nbits)
      settings: AttributesFormatString=Channel: 6, Delay: 61
  detector_block_v27 : Subsystem  AncestorBlock=honestlibrary/detector_block_v2  mask(Basic block for FRB detection){chn=7, lat=69, nbits=4}
      mask prompts: chn "Channel"; lat "Latency"; nbits "Number of Bits (Counter)"
      mask help:
      | Delays a certain channel a number of latency clock cycles, according to the fixed DM table.
      | This version incorporates an internal counter (nbits) to know when store or give a certain value.
      mask init:
      | detector_block_init_v2(gcb,'chn',chn,'lat',lat,'nbits',nbits)
      settings: AttributesFormatString=Channel: 7, Delay: 69
  detector_block_v28 : Subsystem  AncestorBlock=honestlibrary/detector_block_v2  mask(Basic block for FRB detection){chn=8, lat=76, nbits=4}
      mask prompts: chn "Channel"; lat "Latency"; nbits "Number of Bits (Counter)"
      mask help:
      | Delays a certain channel a number of latency clock cycles, according to the fixed DM table.
      | This version incorporates an internal counter (nbits) to know when store or give a certain value.
      mask init:
      | detector_block_init_v2(gcb,'chn',chn,'lat',lat,'nbits',nbits)
      settings: AttributesFormatString=Channel: 8, Delay: 76
  detector_block_v29 : Subsystem  AncestorBlock=honestlibrary/detector_block_v2  mask(Basic block for FRB detection){chn=9, lat=83, nbits=4}
      mask prompts: chn "Channel"; lat "Latency"; nbits "Number of Bits (Counter)"
      mask help:
      | Delays a certain channel a number of latency clock cycles, according to the fixed DM table.
      | This version incorporates an internal counter (nbits) to know when store or give a certain value.
      mask init:
      | detector_block_init_v2(gcb,'chn',chn,'lat',lat,'nbits',nbits)
      settings: AttributesFormatString=Channel: 9, Delay: 83
  Output : Outport
  wires:
  Mux/1 -> Output/1
  detector_block_v215/1(Out1) -> Mux/17
  detector_block_v214/1(Out1) -> Mux/16
  detector_block_v213/1(Out1) -> Mux/15
  detector_block_v212/1(Out1) -> Mux/14
  detector_block_v211/1(Out1) -> Mux/13
  detector_block_v210/1(Out1) -> Mux/12
  detector_block_v29/1(Out1) -> Mux/11
  detector_block_v28/1(Out1) -> Mux/10
  detector_block_v27/1(Out1) -> Mux/9
  detector_block_v26/1(Out1) -> Mux/8
  detector_block_v25/1(Out1) -> Mux/7
  detector_block_v24/1(Out1) -> Mux/6
  detector_block_v23/1(Out1) -> Mux/5
  detector_block_v22/1(Out1) -> Mux/4
  detector_block_v21/1(Out1) -> Mux/3
  detector_block_v2/1(Out1) -> Mux/2
  Counter/1 -> Mux/1
  Valid/1 -> Counter/1, detector_block_v215/2(Valid), detector_block_v214/2(Valid), detector_block_v213/2(Valid), detector_block_v212/2(Valid), detector_block_v211/2(Valid), detector_block_v210/2(Valid), detector_block_v29/2(Valid), detector_block_v28/2(Valid), detector_block_v27/2(Valid), detector_block_v26/2(Valid), detector_block_v25/2(Valid), detector_block_v24/2(Valid), detector_block_v23/2(Valid), detector_block_v22/2(Valid), detector_block_v21/2(Valid), detector_block_v2/2(Valid)
  Data/1 -> detector_block_v215/1(Data), detector_block_v214/1(Data), detector_block_v213/1(Data), detector_block_v212/1(Data), detector_block_v211/1(Data), detector_block_v210/1(Data), detector_block_v29/1(Data), detector_block_v28/1(Data), detector_block_v27/1(Data), detector_block_v26/1(Data), detector_block_v25/1(Data), detector_block_v24/1(Data), detector_block_v23/1(Data), detector_block_v22/1(Data), detector_block_v21/1(Data), detector_block_v2/1(Data)

== system frbd_64ch_600mhz2/Parallel_Dedispersor_v1/Dedispersor_v2_2 ==
  Data : Inport
  Valid : Inport  Port=2
  Counter : xbsIndex_r4/Counter  cnt_type=Free Running  cnt_to=Inf  operation=Up  start_count=0  cnt_by_val=1  arith_type=Unsigned  n_bits=4  bin_pt=0  load_pin=off  rst=off  en=on  explicit_period=on  period=1  dbl_ovrd=off  use_behavioral_HDL=off  implementation=Fabric  block_type=counter
  Mux : xbsIndex_r4/Mux  inputs=16  en=off  latency=0  precision=Full  arith_type=Unsigned  n_bits=16  bin_pt=14  quantization=Truncate  overflow=Wrap  dbl_ovrd=off  block_type=mux
  detector_block_v2 : Subsystem  AncestorBlock=honestlibrary/detector_block_v2  mask(Basic block for FRB detection){chn=0, lat=2, nbits=4}
      mask prompts: chn "Channel"; lat "Latency"; nbits "Number of Bits (Counter)"
      mask help:
      | Delays a certain channel a number of latency clock cycles, according to the fixed DM table.
      | This version incorporates an internal counter (nbits) to know when store or give a certain value.
      mask init:
      | detector_block_init_v2(gcb,'chn',chn,'lat',lat,'nbits',nbits)
      settings: AttributesFormatString=Channel: 0, Delay: 2
  detector_block_v21 : Subsystem  AncestorBlock=honestlibrary/detector_block_v2  mask(Basic block for FRB detection){chn=1, lat=15, nbits=4}
      mask prompts: chn "Channel"; lat "Latency"; nbits "Number of Bits (Counter)"
      mask help:
      | Delays a certain channel a number of latency clock cycles, according to the fixed DM table.
      | This version incorporates an internal counter (nbits) to know when store or give a certain value.
      mask init:
      | detector_block_init_v2(gcb,'chn',chn,'lat',lat,'nbits',nbits)
      settings: AttributesFormatString=Channel: 1, Delay: 15
  detector_block_v210 : Subsystem  AncestorBlock=honestlibrary/detector_block_v2  mask(Basic block for FRB detection){chn=10, lat=90, nbits=4}
      mask prompts: chn "Channel"; lat "Latency"; nbits "Number of Bits (Counter)"
      mask help:
      | Delays a certain channel a number of latency clock cycles, according to the fixed DM table.
      | This version incorporates an internal counter (nbits) to know when store or give a certain value.
      mask init:
      | detector_block_init_v2(gcb,'chn',chn,'lat',lat,'nbits',nbits)
      settings: AttributesFormatString=Channel: 10, Delay: 90
  detector_block_v211 : Subsystem  AncestorBlock=honestlibrary/detector_block_v2  mask(Basic block for FRB detection){chn=11, lat=96, nbits=4}
      mask prompts: chn "Channel"; lat "Latency"; nbits "Number of Bits (Counter)"
      mask help:
      | Delays a certain channel a number of latency clock cycles, according to the fixed DM table.
      | This version incorporates an internal counter (nbits) to know when store or give a certain value.
      mask init:
      | detector_block_init_v2(gcb,'chn',chn,'lat',lat,'nbits',nbits)
      settings: AttributesFormatString=Channel: 11, Delay: 96
  detector_block_v212 : Subsystem  AncestorBlock=honestlibrary/detector_block_v2  mask(Basic block for FRB detection){chn=12, lat=101, nbits=4}
      mask prompts: chn "Channel"; lat "Latency"; nbits "Number of Bits (Counter)"
      mask help:
      | Delays a certain channel a number of latency clock cycles, according to the fixed DM table.
      | This version incorporates an internal counter (nbits) to know when store or give a certain value.
      mask init:
      | detector_block_init_v2(gcb,'chn',chn,'lat',lat,'nbits',nbits)
      settings: AttributesFormatString=Channel: 12, Delay: 101
  detector_block_v213 : Subsystem  AncestorBlock=honestlibrary/detector_block_v2  mask(Basic block for FRB detection){chn=13, lat=106, nbits=4}
      mask prompts: chn "Channel"; lat "Latency"; nbits "Number of Bits (Counter)"
      mask help:
      | Delays a certain channel a number of latency clock cycles, according to the fixed DM table.
      | This version incorporates an internal counter (nbits) to know when store or give a certain value.
      mask init:
      | detector_block_init_v2(gcb,'chn',chn,'lat',lat,'nbits',nbits)
      settings: AttributesFormatString=Channel: 13, Delay: 106
  detector_block_v214 : Subsystem  AncestorBlock=honestlibrary/detector_block_v2  mask(Basic block for FRB detection){chn=14, lat=111, nbits=4}
      mask prompts: chn "Channel"; lat "Latency"; nbits "Number of Bits (Counter)"
      mask help:
      | Delays a certain channel a number of latency clock cycles, according to the fixed DM table.
      | This version incorporates an internal counter (nbits) to know when store or give a certain value.
      mask init:
      | detector_block_init_v2(gcb,'chn',chn,'lat',lat,'nbits',nbits)
      settings: AttributesFormatString=Channel: 14, Delay: 111
  detector_block_v215 : Subsystem  AncestorBlock=honestlibrary/detector_block_v2  mask(Basic block for FRB detection){chn=15, lat=115, nbits=4}
      mask prompts: chn "Channel"; lat "Latency"; nbits "Number of Bits (Counter)"
      mask help:
      | Delays a certain channel a number of latency clock cycles, according to the fixed DM table.
      | This version incorporates an internal counter (nbits) to know when store or give a certain value.
      mask init:
      | detector_block_init_v2(gcb,'chn',chn,'lat',lat,'nbits',nbits)
      settings: AttributesFormatString=Channel: 15, Delay: 115
  detector_block_v22 : Subsystem  AncestorBlock=honestlibrary/detector_block_v2  mask(Basic block for FRB detection){chn=2, lat=26, nbits=4}
      mask prompts: chn "Channel"; lat "Latency"; nbits "Number of Bits (Counter)"
      mask help:
      | Delays a certain channel a number of latency clock cycles, according to the fixed DM table.
      | This version incorporates an internal counter (nbits) to know when store or give a certain value.
      mask init:
      | detector_block_init_v2(gcb,'chn',chn,'lat',lat,'nbits',nbits)
      settings: AttributesFormatString=Channel: 2, Delay: 26
  detector_block_v23 : Subsystem  AncestorBlock=honestlibrary/detector_block_v2  mask(Basic block for FRB detection){chn=3, lat=37, nbits=4}
      mask prompts: chn "Channel"; lat "Latency"; nbits "Number of Bits (Counter)"
      mask help:
      | Delays a certain channel a number of latency clock cycles, according to the fixed DM table.
      | This version incorporates an internal counter (nbits) to know when store or give a certain value.
      mask init:
      | detector_block_init_v2(gcb,'chn',chn,'lat',lat,'nbits',nbits)
      settings: AttributesFormatString=Channel: 3, Delay: 37
  detector_block_v24 : Subsystem  AncestorBlock=honestlibrary/detector_block_v2  mask(Basic block for FRB detection){chn=4, lat=46, nbits=4}
      mask prompts: chn "Channel"; lat "Latency"; nbits "Number of Bits (Counter)"
      mask help:
      | Delays a certain channel a number of latency clock cycles, according to the fixed DM table.
      | This version incorporates an internal counter (nbits) to know when store or give a certain value.
      mask init:
      | detector_block_init_v2(gcb,'chn',chn,'lat',lat,'nbits',nbits)
      settings: AttributesFormatString=Channel: 4, Delay: 46
  detector_block_v25 : Subsystem  AncestorBlock=honestlibrary/detector_block_v2  mask(Basic block for FRB detection){chn=5, lat=55, nbits=4}
      mask prompts: chn "Channel"; lat "Latency"; nbits "Number of Bits (Counter)"
      mask help:
      | Delays a certain channel a number of latency clock cycles, according to the fixed DM table.
      | This version incorporates an internal counter (nbits) to know when store or give a certain value.
      mask init:
      | detector_block_init_v2(gcb,'chn',chn,'lat',lat,'nbits',nbits)
      settings: AttributesFormatString=Channel: 5, Delay: 55
  detector_block_v26 : Subsystem  AncestorBlock=honestlibrary/detector_block_v2  mask(Basic block for FRB detection){chn=6, lat=63, nbits=4}
      mask prompts: chn "Channel"; lat "Latency"; nbits "Number of Bits (Counter)"
      mask help:
      | Delays a certain channel a number of latency clock cycles, according to the fixed DM table.
      | This version incorporates an internal counter (nbits) to know when store or give a certain value.
      mask init:
      | detector_block_init_v2(gcb,'chn',chn,'lat',lat,'nbits',nbits)
      settings: AttributesFormatString=Channel: 6, Delay: 63
  detector_block_v27 : Subsystem  AncestorBlock=honestlibrary/detector_block_v2  mask(Basic block for FRB detection){chn=7, lat=71, nbits=4}
      mask prompts: chn "Channel"; lat "Latency"; nbits "Number of Bits (Counter)"
      mask help:
      | Delays a certain channel a number of latency clock cycles, according to the fixed DM table.
      | This version incorporates an internal counter (nbits) to know when store or give a certain value.
      mask init:
      | detector_block_init_v2(gcb,'chn',chn,'lat',lat,'nbits',nbits)
      settings: AttributesFormatString=Channel: 7, Delay: 71
  detector_block_v28 : Subsystem  AncestorBlock=honestlibrary/detector_block_v2  mask(Basic block for FRB detection){chn=8, lat=78, nbits=4}
      mask prompts: chn "Channel"; lat "Latency"; nbits "Number of Bits (Counter)"
      mask help:
      | Delays a certain channel a number of latency clock cycles, according to the fixed DM table.
      | This version incorporates an internal counter (nbits) to know when store or give a certain value.
      mask init:
      | detector_block_init_v2(gcb,'chn',chn,'lat',lat,'nbits',nbits)
      settings: AttributesFormatString=Channel: 8, Delay: 78
  detector_block_v29 : Subsystem  AncestorBlock=honestlibrary/detector_block_v2  mask(Basic block for FRB detection){chn=9, lat=84, nbits=4}
      mask prompts: chn "Channel"; lat "Latency"; nbits "Number of Bits (Counter)"
      mask help:
      | Delays a certain channel a number of latency clock cycles, according to the fixed DM table.
      | This version incorporates an internal counter (nbits) to know when store or give a certain value.
      mask init:
      | detector_block_init_v2(gcb,'chn',chn,'lat',lat,'nbits',nbits)
      settings: AttributesFormatString=Channel: 9, Delay: 84
  Output : Outport
  wires:
  Mux/1 -> Output/1
  detector_block_v215/1(Out1) -> Mux/17
  detector_block_v214/1(Out1) -> Mux/16
  detector_block_v213/1(Out1) -> Mux/15
  detector_block_v212/1(Out1) -> Mux/14
  detector_block_v211/1(Out1) -> Mux/13
  detector_block_v210/1(Out1) -> Mux/12
  detector_block_v29/1(Out1) -> Mux/11
  detector_block_v28/1(Out1) -> Mux/10
  detector_block_v27/1(Out1) -> Mux/9
  detector_block_v26/1(Out1) -> Mux/8
  detector_block_v25/1(Out1) -> Mux/7
  detector_block_v24/1(Out1) -> Mux/6
  detector_block_v23/1(Out1) -> Mux/5
  detector_block_v22/1(Out1) -> Mux/4
  detector_block_v21/1(Out1) -> Mux/3
  detector_block_v2/1(Out1) -> Mux/2
  Counter/1 -> Mux/1
  Valid/1 -> Counter/1, detector_block_v215/2(Valid), detector_block_v214/2(Valid), detector_block_v213/2(Valid), detector_block_v212/2(Valid), detector_block_v211/2(Valid), detector_block_v210/2(Valid), detector_block_v29/2(Valid), detector_block_v28/2(Valid), detector_block_v27/2(Valid), detector_block_v26/2(Valid), detector_block_v25/2(Valid), detector_block_v24/2(Valid), detector_block_v23/2(Valid), detector_block_v22/2(Valid), detector_block_v21/2(Valid), detector_block_v2/2(Valid)
  Data/1 -> detector_block_v215/1(Data), detector_block_v214/1(Data), detector_block_v213/1(Data), detector_block_v212/1(Data), detector_block_v211/1(Data), detector_block_v210/1(Data), detector_block_v29/1(Data), detector_block_v28/1(Data), detector_block_v27/1(Data), detector_block_v26/1(Data), detector_block_v25/1(Data), detector_block_v24/1(Data), detector_block_v23/1(Data), detector_block_v22/1(Data), detector_block_v21/1(Data), detector_block_v2/1(Data)
